simulink model "linear"  (R2020b)
settings: Solver=VariableStepAuto  StartTime=0.0  StopTime=30  RelTol=1e-3
values from neighbouring files (symbols this model uses):
  A = [0 1 0 ... (first row only)    [linear_calc.m]    (also in setup_sim.m)
  B = [ 0 0 0 ... (first row only)    [linear_calc.m]    (also in setup_sim.m)
  C = pid(2.8446,7.8712,0.02208)    [linear_calc.m]    (also in setup_sim.m = [1 0 0)
libraries: simulink_extras x1
settings Model: Creator=zhans  LastModifiedBy=zhans

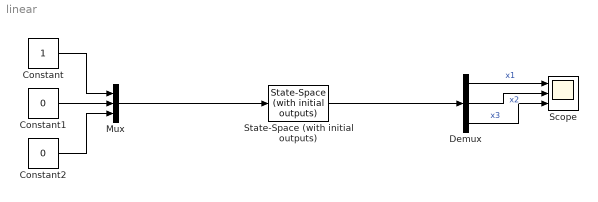
== system linear ==
  Constant : Constant
  Constant1 : Constant  Value=0
  Constant2 : Constant  Value=0
  Demux : Demux  Outputs=3
  Mux : Mux  Inputs=3
  Scope : Scope  NumInputPorts=3
  State-Space (with initial outputs) : simulink_extras/Additional Linear/State-Space (with initial outputs)  A=A  B=B  C=C  D=[ 0 0 0; 0 0 0; 0 0 0]  U0=[0 ; 0 ; 0]  Y0=[0 ; 0 ; 0]
      settings: SourceProductBaseCode=SL
  wires:
  Constant/1 -> Mux/1
  Constant1/1 -> Mux/2
  Constant2/1 -> Mux/3
  Mux/1 -> State-Space (with initial outputs)/1
  State-Space (with initial outputs)/1 -> Demux/1
  Demux/1 -> Scope/1  "x1"
  Demux/2 -> Scope/2  "x2"
  Demux/3 -> Scope/3  "x3"
